simulink model "PF_Simulink_TEST"  (R2022b)
settings: Solver=FixedStepAuto  StartTime=0.0  StopTime=25  FixedStep=0.10  RelTol=1e-3
values from neighbouring files (symbols this model uses):
  D1 = W2_newnew(x0)    [main_S_F.m]
  D2 = W3_newnew(x0)    [main_S_F.m]
  num_particles = 75    [main_S_F.m]
  std_dev1 = std_dev    [main_S_F.m]
  std_dev2 = [1.5; 1.5; 1e-3; 1e-3; 1e-6; 0.2;0.2]    [main_S_F.m]
  W_xu_ranges = [ ... (first row only)    [main_S_F.m]
  W_xucar1 = [10;10;1e-4;1e-4;1e-4;0.50;0.1]    [main_S_F.m]
  W_xucar2 = [10;10;1e-4;1e-4;1e-4;0.50;0.1]    [main_S_F.m]
  x0 = [0;-45;pi/2;0;0;-30;0;0;10;0]    [main_S_F.m]
undefined symbols (not defined in the file or in its folder): estimated_W_xu_car2, estimated_Wxu_car1
(part 2 of 2)

== matlab function PF_Simulink_TEST/Particle Filter 2/PF_pred_trajectories2/OCP_SOLVE_SFunction11/MATLAB Function ==
  data: x0 input; p output; W_xu input; W_xu1 input; testtheta1 input; testtheta2 input; D1 input; D2 input; S1 output; S2 output
function [p, S1, S2] = OCP_prepare_parameters22(x0, W_xu, W_xu1, testtheta1, testtheta2, D1, D2)
    nx = length(x0);
    nu = 4;
    ocp_N = 20; % Number of prediction steps
    % Initialize the parameter array
    p = zeros(504, 1); % 504 elements as per your structure

    % Prepare reference points
    current_state1 = x0(1:2); % Use the updated x0 for car 1
    current_state2 = x0(6:7); % Use the updated x0 for car 2
    
    closest_idx1 = findClosestPoint(current_state1, D1);
    closest_idx2 = findClosestPoint(current_state2, D2);
    
    % Reference points for car 1
    if closest_idx1 + ocp_N <= size(D1, 2)
        reference_points1 = D1(:, closest_idx1:closest_idx1 + ocp_N);
    else
        remaining_points1 = size(D1, 2) - closest_idx1 + 1;
        reference_points1 = D1(:, closest_idx1:end);
        additional_points1 = (ocp_N + 1) - remaining_points1;

        last_x1 = D1(1, end);
        last_y1 = D1(2, end);
        new_x1 = last_x1 - (1:additional_points1) * 0.1; % Assuming 0.1m per step
        new_y1 = last_y1 * ones(1, additional_points1);

        extended_points1 = [new_x1; new_y1];
        reference_points1 = [reference_points1, extended_points1];
    end
    
    % Reference points for car 2
    if closest_idx2 + ocp_N <= size(D2, 2)
        reference_points2 = D2(:, closest_idx2:closest_idx2 + ocp_N);
    else
        remaining_points2 = size(D2, 2) - closest_idx2 + 1;
        reference_points2 = D2(:, closest_idx2:end);
        additional_points2 = (ocp_N + 1) - remaining_points2;

        last_x2 = D2(1, end);
        last_y2 = D2(2, end);
        new_x2 = last_x2 + (1:additional_points2) * 0.1; % Assuming 0.1m per step
        new_y2 = last_y2 * ones(1, additional_points2);

        extended_points2 = [new_x2; new_y2];
        reference_points2 = [reference_points2, extended_points2];
    end

    % Create x_traj_init with the specified structure
    x_traj_init = [
        reference_points1; % x1, y1, ...
        testtheta1';       % theta1
        zeros(1, ocp_N + 1); % v1
        zeros(1, ocp_N + 1); % s1
        reference_points2; % x2, y2, ...
        testtheta2';       % theta2
        zeros(1, ocp_N + 1); % v2
        zeros(1, ocp_N + 1)  % s2
    ];

    % Check sizes
    S1 = size(x_traj_init, 1); % Number of rows
    S2 = size(x_traj_init, 2); % Number of columns

%     % Ensure that x_traj_init has enough rows
%     if S1 < 20
%         error('x_traj_init does not have enough rows. Current size: %d', S1);
%     end

    % Fill the parameter array with references and weights
    for jj = 0:ocp_N
        % Fill references for the first car
        p((jj) * (10 + 14) + 1:(jj) * (10 + 14) + 5) = x_traj_init(1:5, jj + 1); % Ref for car 1
        
        % Fill references for the second car
        p((jj) * (10 + 14) + 6:(jj) * (10 + 14) + 10) = x_traj_init(6:10, jj + 1); % Ref for car 2
        
        % Fill weights for the first car
        p((jj) * (10 + 14) + 11:(jj) * (10 + 14) + 15) = W_xu1(1:5); % Weights for car 1
        
        % Fill weights for the second car
        p((jj) * (10 + 14) + 16:(jj) * (10 + 14) + 20) = W_xu(1:5); % Weights for car 2
        
        % Fill weights for the control inputs
%         p((jj) * (10 + 14) + 21:(jj) * (10 + 14) + 24) = [W_xu(6:7);W_xu1(6:7)]; % Control input weights (4 elements)
        p((jj) * (10 + 14) + 21:(jj) * (10 + 14) + 24) = [W_xu1(6:7);W_xu(6:7)]; % Control input weights (4 elements)
    end

    % Check if the size of p is correct
    assert(length(p) == 504, 'Parameter array must have 504 elements.');

    % Output parameter array
end

== matlab function PF_Simulink_TEST/Particle Filter 2/PF_pred_trajectories2/OCP_SOLVE_SFunction11/MATLAB Function1 ==
  data: lbu output
function lbu = LBU
% Define lower bounds for control inputs
lbu_control = [-11.5; -1; -11.5; -1]; % Control inputs

% Determine how many times to repeat the control bounds
num_repeats = ceil(80 / length(lbu_control)); % Calculate how many times to repeat
lbu = repmat(lbu_control, num_repeats, 1); % Repeat to create a long enough array
lbu = lbu(1:80); % Truncate to exactly 80 elements

% Check size
assert(length(lbu) == 80, 'Lower bounds array must have 80 elements.');

end

== matlab function PF_Simulink_TEST/Particle Filter 2/PF_pred_trajectories2/OCP_SOLVE_SFunction11/MATLAB Function2 ==
  data: ubu output
function ubu = UBU
% Define lower bounds for control inputs
ubu_control = [+11.5; 1; 11.5; 1]; % Control inputs

% Determine how many times to repeat the control bounds
num_repeats = ceil(80 / length(ubu_control)); % Calculate how many times to repeat
ubu = repmat(ubu_control, num_repeats, 1); % Repeat to create a long enough array
ubu = ubu(1:80); % Truncate to exactly 80 elements

% Check size
assert(length(ubu) == 80, 'Lower bounds array must have 80 elements.');

end

== matlab function PF_Simulink_TEST/OCP REFERENCE GENERATOR ==
  data: x0 input; p output; W_xu input; W_xu1 input; testtheta1 input; testtheta2 input; D1 input; D2 input; S1 output; S2 output
function [p, S1, S2] = OCP_prepare_parameters(x0, W_xu, W_xu1, testtheta1, testtheta2, D1, D2)
    nx = length(x0);
    nu = 4;
    ocp_N = 20; % Number of prediction steps
    % Initialize the parameter array
    p = zeros(504, 1); % 504 elements as per your structure

    % Prepare reference points
    current_state1 = x0(1:2); % Use the updated x0 for car 1
    current_state2 = x0(6:7); % Use the updated x0 for car 2
    
    closest_idx1 = findClosestPoint(current_state1, D1);
    closest_idx2 = findClosestPoint(current_state2, D2);
    
    % Reference points for car 1
    if closest_idx1 + ocp_N <= size(D1, 2)
        reference_points1 = D1(:, closest_idx1:closest_idx1 + ocp_N);
    else
        remaining_points1 = size(D1, 2) - closest_idx1 + 1;
        reference_points1 = D1(:, closest_idx1:end);
        additional_points1 = (ocp_N + 1) - remaining_points1;

        last_x1 = D1(1, end);
        last_y1 = D1(2, end);
        new_x1 = last_x1 - (1:additional_points1) * 0.1; % Assuming 0.1m per step
        new_y1 = last_y1 * ones(1, additional_points1);

        extended_points1 = [new_x1; new_y1];
        reference_points1 = [reference_points1, extended_points1];
    end
    
    % Reference points for car 2
    if closest_idx2 + ocp_N <= size(D2, 2)
        reference_points2 = D2(:, closest_idx2:closest_idx2 + ocp_N);
    else
        remaining_points2 = size(D2, 2) - closest_idx2 + 1;
        reference_points2 = D2(:, closest_idx2:end);
        additional_points2 = (ocp_N + 1) - remaining_points2;

        last_x2 = D2(1, end);
        last_y2 = D2(2, end);
        new_x2 = last_x2 + (1:additional_points2) * 0.1; % Assuming 0.1m per step
        new_y2 = last_y2 * ones(1, additional_points2);

        extended_points2 = [new_x2; new_y2];
        reference_points2 = [reference_points2, extended_points2];
    end

    % Create x_traj_init with the specified structure
    x_traj_init = [
        reference_points1; % x1, y1, ...
        testtheta1';       % theta1
        zeros(1, ocp_N + 1); % v1
        zeros(1, ocp_N + 1); % s1
        reference_points2; % x2, y2, ...
        testtheta2';       % theta2
        zeros(1, ocp_N + 1); % v2
        zeros(1, ocp_N + 1)  % s2
    ];

    % Check sizes
    S1 = size(x_traj_init, 1); % Number of rows
    S2 = size(x_traj_init, 2); % Number of columns

%     % Ensure that x_traj_init has enough rows
%     if S1 < 20
%         error('x_traj_init does not have enough rows. Current size: %d', S1);
%     end

    % Fill the parameter array with references and weights
    for jj = 0:ocp_N
        % Fill references for the first car
        p((jj) * (10 + 14) + 1:(jj) * (10 + 14) + 5) = x_traj_init(1:5, jj + 1); % Ref for car 1
        
        % Fill references for the second car
        p((jj) * (10 + 14) + 6:(jj) * (10 + 14) + 10) = x_traj_init(6:10, jj + 1); % Ref for car 2
        
        % Fill weights for the first car
        p((jj) * (10 + 14) + 11:(jj) * (10 + 14) + 15) = W_xu1(1:5); % Weights for car 1
        
        % Fill weights for the second car
        p((jj) * (10 + 14) + 16:(jj) * (10 + 14) + 20) = W_xu(1:5); % Weights for car 2
        
        % Fill weights for the control inputs
%         p((jj) * (10 + 14) + 21:(jj) * (10 + 14) + 24) = [W_xu(6:7);W_xu1(6:7)]; % Control input weights (4 elements)
        p((jj) * (10 + 14) + 21:(jj) * (10 + 14) + 24) = [W_xu1(6:7);W_xu(6:7)]; % Control input weights (4 elements)
    end

    % Check if the size of p is correct
    assert(length(p) == 504, 'Parameter array must have 504 elements.');

    % Output parameter array
end

== matlab function PF_Simulink_TEST/Particle Filter 2/Particles initialization1 ==
  data: num_particles2 input; W_xu_particles2 output size=[num_particles, 7] [..100000]; W_xu_ranges2 input; initial_guess2 input; range_factor2 input; std_dev2 input; weights2 output size=[num_particles,1] [-1..10]
function [W_xu_particles2,weights2] = initializeParticles2(num_particles2, W_xu_ranges2,initial_guess2,range_factor2,std_dev2)
    num_ranges = size(W_xu_ranges2, 1);  % Number of parameters
    W_xu_particles2 = zeros(num_particles2, num_ranges);

    std_dev2=std_dev2*range_factor2;

    
    for i = 1:num_ranges
        % Define the mean and standard deviation for the Gaussian distribution for parameter i
        mean_value = initial_guess2(i);    % Mean for the Gaussian distribution
        std_deviation = std_dev2(i);          % Standard deviation for the Gaussian distribution

        % Generate random particles from a Gaussian distribution
        W_xu_particles2(:, i) = mean_value + std_deviation * randn(num_particles2, 1);
        
        % Clip values to be within the specified range
        W_xu_particles2(:, i) = max(W_xu_ranges2(i, 1), min(W_xu_ranges2(i, 2), W_xu_particles2(:, i)));
    end
    %%% make the x and y the same since we have that knowledge (testing this)
    W_xu_particles2(:,2)=W_xu_particles2(:,1);
    %%%
    
    % Initialize weights uniformly
    weights2 = ones(num_particles2, 1) / num_particles2;
%     
%     particles.W_xu = W_xu_particles;
%     particles.weights = weights;
end

== matlab function PF_Simulink_TEST/MATLAB Function2 ==
  data: ubu output
function ubu = UBU
% Define lower bounds for control inputs
ubu_control = [+11.5; 1; 11.5; 1]; % Control inputs

% Determine how many times to repeat the control bounds
num_repeats = ceil(80 / length(ubu_control)); % Calculate how many times to repeat
ubu = repmat(ubu_control, num_repeats, 1); % Repeat to create a long enough array
ubu = ubu(1:80); % Truncate to exactly 80 elements

% Check size
assert(length(ubu) == 80, 'Lower bounds array must have 80 elements.');

end

== matlab function PF_Simulink_TEST/Reference Generator ==
  data: x0 input; p output; W_xu input; W_xu1 input; testtheta1 input; testtheta2 input; D1 input; D2 input; S1 output; S2 output
function [p, S1, S2] = OCP_prepare_parameters(x0, W_xu, W_xu1, testtheta1, testtheta2, D1, D2)
    nx = length(x0);
    nu = 4;
    ocp_N = 20; % Number of prediction steps
    % Initialize the parameter array
    p = zeros(504, 1); % 504 elements as per your structure

    % Prepare reference points
    current_state1 = x0(1:2); % Use the updated x0 for car 1
    current_state2 = x0(6:7); % Use the updated x0 for car 2
    
    closest_idx1 = findClosestPoint(current_state1, D1);
    closest_idx2 = findClosestPoint(current_state2, D2);
    
    % Reference points for car 1
    if closest_idx1 + ocp_N <= size(D1, 2)
        reference_points1 = D1(:, closest_idx1:closest_idx1 + ocp_N);
    else
        remaining_points1 = size(D1, 2) - closest_idx1 + 1;
        reference_points1 = D1(:, closest_idx1:end);
        additional_points1 = (ocp_N + 1) - remaining_points1;

        last_x1 = D1(1, end);
        last_y1 = D1(2, end);
        new_x1 = last_x1 - (1:additional_points1) * 0.1; % Assuming 0.1m per step
        new_y1 = last_y1 * ones(1, additional_points1);

        extended_points1 = [new_x1; new_y1];
        reference_points1 = [reference_points1, extended_points1];
    end
    
    % Reference points for car 2
    if closest_idx2 + ocp_N <= size(D2, 2)
        reference_points2 = D2(:, closest_idx2:closest_idx2 + ocp_N);
    else
        remaining_points2 = size(D2, 2) - closest_idx2 + 1;
        reference_points2 = D2(:, closest_idx2:end);
        additional_points2 = (ocp_N + 1) - remaining_points2;

        last_x2 = D2(1, end);
        last_y2 = D2(2, end);
        new_x2 = last_x2 + (1:additional_points2) * 0.1; % Assuming 0.1m per step
        new_y2 = last_y2 * ones(1, additional_points2);

        extended_points2 = [new_x2; new_y2];
        reference_points2 = [reference_points2, extended_points2];
    end

    % Create x_traj_init with the specified structure
    x_traj_init = [
        reference_points1; % x1, y1, ...
        testtheta1';       % theta1
        zeros(1, ocp_N + 1); % v1
        zeros(1, ocp_N + 1); % s1
        reference_points2; % x2, y2, ...
        testtheta2';       % theta2
        zeros(1, ocp_N + 1); % v2
        zeros(1, ocp_N + 1)  % s2
    ];

    % Check sizes
    S1 = size(x_traj_init, 1); % Number of rows
    S2 = size(x_traj_init, 2); % Number of columns

%     % Ensure that x_traj_init has enough rows
%     if S1 < 20
%         error('x_traj_init does not have enough rows. Current size: %d', S1);
%     end

    % Fill the parameter array with references and weights
    for jj = 0:ocp_N
        % Fill references for the first car
        p((jj) * (10 + 14) + 1:(jj) * (10 + 14) + 5) = x_traj_init(1:5, jj + 1); % Ref for car 1
        
        % Fill references for the second car
        p((jj) * (10 + 14) + 6:(jj) * (10 + 14) + 10) = x_traj_init(6:10, jj + 1); % Ref for car 2
        
        % Fill weights for the first car
        p((jj) * (10 + 14) + 11:(jj) * (10 + 14) + 15) = W_xu1(1:5); % Weights for car 1
        
        % Fill weights for the second car
        p((jj) * (10 + 14) + 16:(jj) * (10 + 14) + 20) = W_xu(1:5); % Weights for car 2
        
        % Fill weights for the control inputs
%         p((jj) * (10 + 14) + 21:(jj) * (10 + 14) + 24) = [W_xu(6:7);W_xu1(6:7)]; % Control input weights (4 elements)
        p((jj) * (10 + 14) + 21:(jj) * (10 + 14) + 24) = [W_xu1(6:7);W_xu(6:7)]; % Control input weights (4 elements)
    end

    % Check if the size of p is correct
    assert(length(p) == 504, 'Parameter array must have 504 elements.');

    % Output parameter array
end

== matlab function PF_Simulink_TEST/MATLAB Function4 ==
  data: lbu output
function lbu = LBU
% Define lower bounds for control inputs
lbu_control = [-11.5; -1; -11.5; -1]; % Control inputs

% Determine how many times to repeat the control bounds
num_repeats = ceil(80 / length(lbu_control)); % Calculate how many times to repeat
lbu = repmat(lbu_control, num_repeats, 1); % Repeat to create a long enough array
lbu = lbu(1:80); % Truncate to exactly 80 elements

% Check size
assert(length(lbu) == 80, 'Lower bounds array must have 80 elements.');

end

== matlab function PF_Simulink_TEST/MATLAB Function5 ==
  data: ubu output
function ubu = UBU
% Define lower bounds for control inputs
ubu_control = [+11.5; 1; 11.5; 1]; % Control inputs

% Determine how many times to repeat the control bounds
num_repeats = ceil(80 / length(ubu_control)); % Calculate how many times to repeat
ubu = repmat(ubu_control, num_repeats, 1); % Repeat to create a long enough array
ubu = ubu(1:80); % Truncate to exactly 80 elements

% Check size
assert(length(ubu) == 80, 'Lower bounds array must have 80 elements.');

end

== matlab function PF_Simulink_TEST/Particle FIlter 1/PF_pred_trajectories/OCP_SOLVE_SFunction/MATLAB Function ==
  data: x0 input; p output; W_xu input; W_xu1 input; testtheta1 input; testtheta2 input; D1 input; D2 input; S1 output; S2 output
function [p, S1, S2] = OCP_prepare_parameters(x0, W_xu, W_xu1, testtheta1, testtheta2, D1, D2)
    nx = length(x0);
    nu = 4;
    ocp_N = 20; % Number of prediction steps
    % Initialize the parameter array
    p = zeros(504, 1); % 504 elements as per your structure

    % Prepare reference points
    current_state1 = x0(1:2); % Use the updated x0 for car 1
    current_state2 = x0(6:7); % Use the updated x0 for car 2
    
    closest_idx1 = findClosestPoint(current_state1, D1);
    closest_idx2 = findClosestPoint(current_state2, D2);
    
    % Reference points for car 1
    if closest_idx1 + ocp_N <= size(D1, 2)
        reference_points1 = D1(:, closest_idx1:closest_idx1 + ocp_N);
    else
        remaining_points1 = size(D1, 2) - closest_idx1 + 1;
        reference_points1 = D1(:, closest_idx1:end);
        additional_points1 = (ocp_N + 1) - remaining_points1;

        last_x1 = D1(1, end);
        last_y1 = D1(2, end);
        new_x1 = last_x1 - (1:additional_points1) * 0.1; % Assuming 0.1m per step
        new_y1 = last_y1 * ones(1, additional_points1);

        extended_points1 = [new_x1; new_y1];
        reference_points1 = [reference_points1, extended_points1];
    end
    
    % Reference points for car 2
    if closest_idx2 + ocp_N <= size(D2, 2)
        reference_points2 = D2(:, closest_idx2:closest_idx2 + ocp_N);
    else
        remaining_points2 = size(D2, 2) - closest_idx2 + 1;
        reference_points2 = D2(:, closest_idx2:end);
        additional_points2 = (ocp_N + 1) - remaining_points2;

        last_x2 = D2(1, end);
        last_y2 = D2(2, end);
        new_x2 = last_x2 + (1:additional_points2) * 0.1; % Assuming 0.1m per step
        new_y2 = last_y2 * ones(1, additional_points2);

        extended_points2 = [new_x2; new_y2];
        reference_points2 = [reference_points2, extended_points2];
    end

    % Create x_traj_init with the specified structure
    x_traj_init = [
        reference_points1; % x1, y1, ...
        testtheta1';       % theta1
        zeros(1, ocp_N + 1); % v1
        zeros(1, ocp_N + 1); % s1
        reference_points2; % x2, y2, ...
        testtheta2';       % theta2
        zeros(1, ocp_N + 1); % v2
        zeros(1, ocp_N + 1)  % s2
    ];

    % Check sizes
    S1 = size(x_traj_init, 1); % Number of rows
    S2 = size(x_traj_init, 2); % Number of columns

%     % Ensure that x_traj_init has enough rows
%     if S1 < 20
%         error('x_traj_init does not have enough rows. Current size: %d', S1);
%     end

    % Fill the parameter array with references and weights
    for jj = 0:ocp_N
        % Fill references for the first car
        p((jj) * (10 + 14) + 1:(jj) * (10 + 14) + 5) = x_traj_init(1:5, jj + 1); % Ref for car 1
        
        % Fill references for the second car
        p((jj) * (10 + 14) + 6:(jj) * (10 + 14) + 10) = x_traj_init(6:10, jj + 1); % Ref for car 2
        
        % Fill weights for the first car
        p((jj) * (10 + 14) + 11:(jj) * (10 + 14) + 15) = W_xu1(1:5); % Weights for car 1
        
        % Fill weights for the second car
        p((jj) * (10 + 14) + 16:(jj) * (10 + 14) + 20) = W_xu(1:5); % Weights for car 2
        
        % Fill weights for the control inputs
%         p((jj) * (10 + 14) + 21:(jj) * (10 + 14) + 24) = [W_xu(6:7);W_xu1(6:7)]; % Control input weights (4 elements)
        p((jj) * (10 + 14) + 21:(jj) * (10 + 14) + 24) = [W_xu1(6:7);W_xu(6:7)]; % Control input weights (4 elements)

    end

    % Check if the size of p is correct
    assert(length(p) == 504, 'Parameter array must have 504 elements.');

    % Output parameter array
end

== matlab function PF_Simulink_TEST/Particle FIlter 1/PF_pred_trajectories/OCP_SOLVE_SFunction/MATLAB Function1 ==
  data: lbu output
function lbu = LBU
% Define lower bounds for control inputs
lbu_control = [-11.5; -1; -11.5; -1]; % Control inputs

% Determine how many times to repeat the control bounds
num_repeats = ceil(80 / length(lbu_control)); % Calculate how many times to repeat
lbu = repmat(lbu_control, num_repeats, 1); % Repeat to create a long enough array
lbu = lbu(1:80); % Truncate to exactly 80 elements

% Check size
assert(length(lbu) == 80, 'Lower bounds array must have 80 elements.');

end

== matlab function PF_Simulink_TEST/Particle FIlter 1/PF_pred_trajectories/OCP_SOLVE_SFunction/MATLAB Function2 ==
  data: ubu output
function ubu = UBU
% Define lower bounds for control inputs
ubu_control = [+11.5; 1; 11.5; 1]; % Control inputs

% Determine how many times to repeat the control bounds
num_repeats = ceil(80 / length(ubu_control)); % Calculate how many times to repeat
ubu = repmat(ubu_control, num_repeats, 1); % Repeat to create a long enough array
ubu = ubu(1:80); % Truncate to exactly 80 elements

% Check size
assert(length(ubu) == 80, 'Lower bounds array must have 80 elements.');

end

== matlab function PF_Simulink_TEST/Particle FIlter 1/PF_pred_trajectories/MATLAB Function ==
  data: u input; Y output size=[14,num_particles]; i input
function Y = fcn(u, i)
    persistent Y_storage; % Declare Y_storage as a persistent variable

    if isempty(Y_storage) % Initialize on the first call
        Y_storage = []; % Initialize as an empty array
    end

    if i == 1
        Y_storage = u; % Assign the first input directly
    else
        Y_storage = [Y_storage u]; % Concatenate the new input
    end

    Y = Y_storage; % Output the accumulated results
end
